simulink model "lastsim"  (R2022b)
settings: Solver=VariableStepAuto  StartTime=0.0  StopTime=10.0  RelTol=1e-3
undefined symbols (not defined in the file or in its folder): d_a, d_r, d_t, d_y, T_s, wt
libraries: cstblocks x2, simulink x1
settings Model: Creator=melis  LastModifiedBy=franc
settings DataIOCC: ReturnWorkspaceOutputs=off
settings DebuggingCC: UnconnectedInputMsg=warning  UnconnectedOutputMsg=warning  UnconnectedLineMsg=warning
settings ModelReferenceCC: EnableRefExpFcnMdlSchedulingChecks=on
settings RTWCC: DLArmComputeVersion=19.05

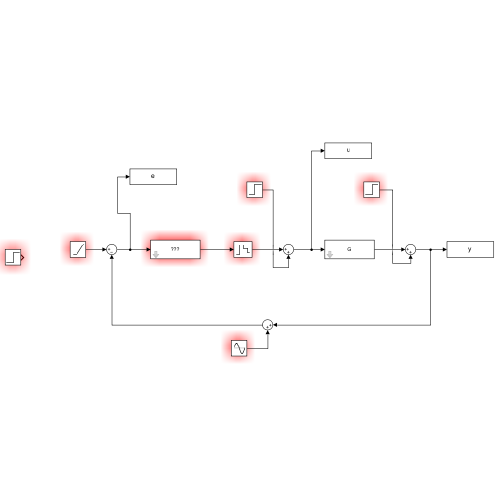
[thumbnail: Simulink's stored preview of the top-level diagram]
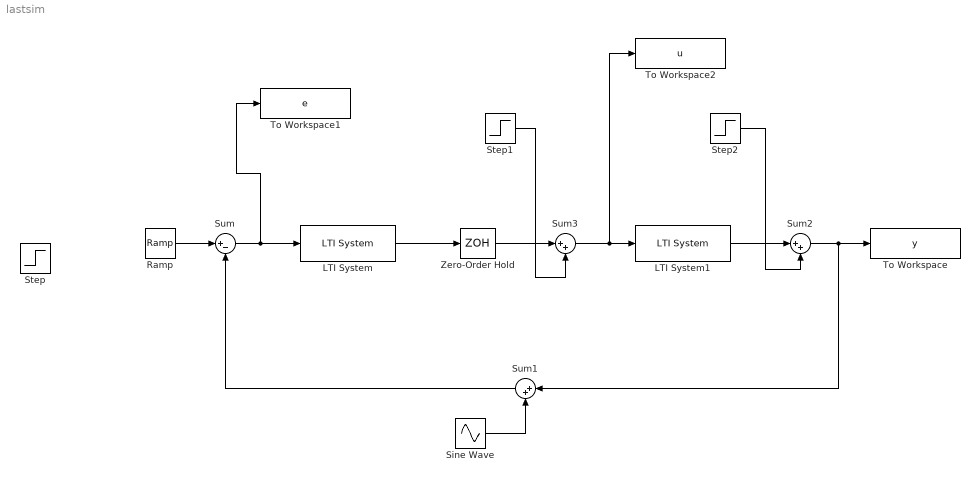
== system lastsim ==
  LTI System : cstblocks/LTI System  sys=C_d  IC=[]
  LTI System1 : cstblocks/LTI System  sys=G  IC=[]
  Ramp : simulink/Sources/Ramp  slope=d_r  start=0  InitialOutput=0
  Sine Wave : Sin  Amplitude=d_t  Frequency=wt  SampleTime=0
  Step : Step  Time=0  After=d_r  SampleTime=0
  Step1 : Step  Time=0  After=d_a  SampleTime=0
  Step2 : Step  Time=0  After=d_y  SampleTime=0
  Sum : Sum  Inputs=|+-
  Sum1 : Sum  Inputs=|++
  Sum2 : Sum  Inputs=|++
  Sum3 : Sum  Inputs=|++
  To Workspace : ToWorkspace  VariableName=y  SaveFormat=Timeseries  SampleTime=-1
  To Workspace1 : ToWorkspace  VariableName=e  SaveFormat=Timeseries  SampleTime=-1
  To Workspace2 : ToWorkspace  VariableName=u  SaveFormat=Timeseries  SampleTime=-1
  Zero-Order Hold : ZeroOrderHold  SampleTime=T_s
  wires:
  Sum/1 -> To Workspace1/1, LTI System/1
  Step1/1 -> Sum3/2
  LTI System/1 -> Zero-Order Hold/1
  Zero-Order Hold/1 -> Sum3/1
  Sum3/1 -> To Workspace2/1, LTI System1/1
  Step2/1 -> Sum2/2
  LTI System1/1 -> Sum2/1
  Sum2/1 -> Sum1/1, To Workspace/1
  Sine Wave/1 -> Sum1/2
  Sum1/1 -> Sum/2
  Ramp/1 -> Sum/1
